simulink model "Udan_SOC"  (R2017b)
settings: Solver=FixedStepAuto  StartTime=0.0  StopTime=1000  FixedStep=0.1  RelTol=1e-3
values from neighbouring files (symbols this model uses):
  DenominatorOfIntegratorFactor = 100.0    [SOC_Stateflow.sldd]
  SOC_CalcSohLKT = 1.0    [SOC_Stateflow.sldd]
  SOC_CalcSOHTempLimit = 70.0    [SOC_Stateflow.sldd]
  SOC_CapPerCycle = 100.0    [SOC_Stateflow.sldd]
  SOC_CapTemp_HLimit = 200.0    [SOC_Stateflow.sldd]
  SOC_CapTemp_LLimit = 0.0    [SOC_Stateflow.sldd]
  Soc_ConfigInfo = 0    [SOC_Stateflow.sldd]
  SOC_DchgEndCalib = 0.0    [SOC_Stateflow.sldd]
  SOC_DiffVoltMin = 10.0    [SOC_Stateflow.sldd]
  SOC_DSOCJumpMax = 500.0    [SOC_Stateflow.sldd]
  SOC_EfficientHighLimit = 250.0    [SOC_Stateflow.sldd]
  SOC_EfficientLowLimit = 40.0    [SOC_Stateflow.sldd]
  SOC_EmptyAus = 0.0    [SOC_Stateflow.sldd]
  SOC_EnableOcv = 1.0    [SOC_Stateflow.sldd]
  SOC_END_CALIB_STATE : value not decoded    [SOC_Stateflow.sldd]
  SOC_HighRealSoc = 95.0    [SOC_Stateflow.sldd]
  SOC_LKTSohCycles = 0.0 1.0 10.0 20.0 30.0 40.0 50.0 60.0 70.0 80.0 90.0 100.0 110.0 120.0 130.0 140.0 150.0 160.0 170.0 180.0 190.0 200.0 210.0 220.0 230.0 240.0 250.0 260.0 270.0 280.0 290.0 300.0 310.0 320.0 330.0 340.0 350.0 360.0 370.0 380.0 390.0 400.0 410.0 420.0 430.0 440.0 450.0 460.0 470.0 480.0 490.0 500.0 510.0 520.0 530.0 540.0 550.0 560.0 570.0 580.0 590.0 600.0 610.0 620.0 630.0 640.0 650.0 660.0 670.0    [SOC_Stateflow.sldd]
  SOC_LKTSohTable = 1000.0 991.0 989.0 992.0 993.0 995.0 994.0 993.0 1000.0 997.0 1002.0 1000.0 992.0 1000.0 989.0 992.0 989.0 994.0 989.0 993.0 994.0 994.0 994.0 993.0 991.0 991.0 992.0 993.0 991.0 985.0 985.0 985.0 979.0 975.0 978.0 984.0 982.0 974.0 975.0 972.0 972.0 975.0 977.0 977.0 974.0 971.0 973.0 971.0 966.0 968.0 965.0 959.0 957.0 956.0 957.0 954.0 955.0 951.0 954.0 951.0 942.0 942.0 940.0 942.0 947.0 949.0    [SOC_Stateflow.sldd]
  SOC_LowRealSoc = 5.0    [SOC_Stateflow.sldd]
  SOC_NominalCap_AmS = 576000000.0    [SOC_Stateflow.sldd]
  SOC_NominalVol = 4000.0    [SOC_Stateflow.sldd]
  SOC_OCVTemp_HLimit = 106.0    [SOC_Stateflow.sldd]
  SOC_OCVTemp_LLimit = 29.0    [SOC_Stateflow.sldd]
  SOC_ShortCalibDSoc = 1.0    [SOC_Stateflow.sldd]
  SOC_SOCResolution = 10000.0    [SOC_Stateflow.sldd]
  SOC_SohCalcCapPercent = 8.0    [SOC_Stateflow.sldd]
  SOC_SohCalcHighLimit = 60.0    [SOC_Stateflow.sldd]
  SOC_SohCalcLowLimit = 10.0    [SOC_Stateflow.sldd]
  SOC_SohCalcMidLimit = 30.0    [SOC_Stateflow.sldd]
  SOC_SOHResolution = 1000.0    [SOC_Stateflow.sldd]
  SOC_State = <binary blob, 1163 chars, not shown>    [SOC_Stateflow.sldd]
  SOC_TempCap_CapBuffer : value not decoded    [SOC_Stateflow.sldd]
  SOC_TempCap_TempBuffer : value not decoded    [SOC_Stateflow.sldd]
  SocOcvCalib_ConfigInfo = 0.0    [SOC_Stateflow.sldd]
  SocOcvCalib_SocBuffer1 : value not decoded    [SOC_Stateflow.sldd]
  SocOcvCalib_TempBuffer : value not decoded    [SOC_Stateflow.sldd]
  SocOcvCalib_VoltageBuffer1 = 3300.0 3303.0 3305.0 3307.0 3310.0 3311.0 3313.0 3314.0 3316.0 3317.0 3319.0 3320.0 3322.0 3323.0 3325.0 3322.0 3323.0 3325.0 3310.0 3313.0 3315.0 3317.0 3320.0 3321.0 3323.0 3324.0 3326.0 3327.0 3329.0 3330.0 3332.0 3333.0 3335.0 3332.0 3333.0 3335.0 3320.0 3323.0 3325.0 3327.0 3330.0 3331.0 3333.0 3334.0 3336.0 3337.0 3339.0 3340.0 3342.0 3343.0 3345.0 3342.0 3343.0 3345.0 3330.0 3333.0 3335.0 3    [SOC_Stateflow.sldd]
  SOHCalibCycle = 10.0    [SOC_Stateflow.sldd]
undefined symbols (not defined in the file or in its folder): DatetimeM_GetReturnType, ParameterM_EeepParaIndexType, Soc_CumuLativeTypeType, SOC_EgthTempChgValue, Soc_EnergyBuffer, SOC_FithTempChgValue, SOC_FstSlowTempChgValue, SOC_FstTempChgValue, SOC_FthTempChgValue, SOC_MaxCap_AmS, SOC_SethTempChgValue, SOC_SixTempChgValue, SOC_SndSlowTempChgValue, SOC_SndTempChgValue, SOC_TrdSlowTempChgValue, SOC_TrdTempChgValue, SocDiagCalib_NoCalibReasonType
libraries: simulink x138, hdlsllib x24, dspindex x4
(part 6 of 10)

== system Udan_SOC/SOC_Calculate/UdanSOCCalcn/CalcnLeftChargeTime/CalcLeftTime1 ==
  DLeftCap : Inport
  LowTemp : Inport  Port=2
  PackCur : Inport  Port=3
  TotalCap : Inport  Port=4
  HighTemp : Inport  Port=5
  Enable : EnablePort
  Bus Selector : BusSelector  OutputSignals=FstDecreaseCur,SndDecreaseCur,TrdDecreaseCur,LstDecreaseCur
  Bus Selector1 : BusSelector  OutputSignals=FstDecreaseCur,SndDecreaseCur,TrdDecreaseCur,LstDecreaseCur
  CalcLeftTime : Stateflow chart  TreatAsAtomicUnit=on
  Constant : Constant  Value=9490  OutDataTypeStr=uint16
  Constant1 : Constant  Value=9000  OutDataTypeStr=uint16
  Constant10 : Constant  Value=SOC_SOCResolution  OutDataTypeStr=uint16
  Constant11 : Constant  Value=65535  OutDataTypeStr=uint32
  Constant2 : Constant  Value=9500  OutDataTypeStr=uint16
  Constant3 : Constant  Value=SOC_FstSlowTempChgValue  OutDataTypeStr=Bus: SOC_ChgCurrentType
  Constant4 : Constant  Value=SOC_FstSlowTempChgValue  OutDataTypeStr=Bus: SOC_ChgCurrentType
  Constant5 : Constant  Value=SOC_SndSlowTempChgValue  OutDataTypeStr=Bus: SOC_ChgCurrentType
  Constant6 : Constant  Value=SOC_TrdSlowTempChgValue  OutDataTypeStr=Bus: SOC_ChgCurrentType
  Constant7 : Constant  Value=SOC_SndSlowTempChgValue  OutDataTypeStr=Bus: SOC_ChgCurrentType
  Constant8 : Constant  Value=SOC_TrdSlowTempChgValue  OutDataTypeStr=Bus: SOC_ChgCurrentType
  Constant9 : Constant  Value=65535  OutDataTypeStr=uint32
  Divide : Product  Inputs=*/*  OutDataTypeStr=uint32
  Divide1 : Product  Inputs=*/*  OutDataTypeStr=uint32
  Divide2 : Product  Inputs=*/*  OutDataTypeStr=uint32
  MinMax{,1..3} (4 alike) : MinMax  Inputs=2
  SelectChgCurrent : Stateflow chart  TreatAsAtomicUnit=on
  SelectChgCurrent1 : Stateflow chart  TreatAsAtomicUnit=on
  Terminator : Terminator
  Terminator1 : Terminator
  LeftChargeTime : Outport
  PackCurOk : Outport  Port=2
  wires:
  Constant/1 -> Divide/3
  Constant1/1 -> Divide1/3
  Constant10/1 -> Divide2/2, Divide1/2, Divide/2
  Constant2/1 -> Divide2/3
  LowTemp/1 -> SelectChgCurrent/1(BatTemp)
  Constant4/1 -> SelectChgCurrent/2(FstChgCur)
  Constant5/1 -> SelectChgCurrent/3(SndChgCur)
  Constant6/1 -> SelectChgCurrent/4(TrdChgCur)
  SelectChgCurrent/1(ChgCurOut) -> Bus Selector/1
  DLeftCap/1 -> CalcLeftTime/1(DleftCap)
  TotalCap/1 -> CalcLeftTime/3(NominalCap), Divide2/1, Divide1/1, Divide/1
  Divide/1 -> CalcLeftTime/4(FstDecPnt)
  Constant9/1 -> CalcLeftTime/5(SndDecPnt)
  Constant11/1 -> CalcLeftTime/6(TrdDecPnt)
  MinMax/1 -> CalcLeftTime/7(Cur1)
  MinMax1/1 -> CalcLeftTime/8(Cur2)
  MinMax2/1 -> CalcLeftTime/9(Cur3)
  MinMax3/1 -> CalcLeftTime/10(Cur4)
  CalcLeftTime/1(TimeOut) -> LeftChargeTime/1
  PackCur/1 -> CalcLeftTime/2(PackCur)
  CalcLeftTime/2(result) -> PackCurOk/1
  Constant8/1 -> SelectChgCurrent1/4(TrdChgCur)
  Constant3/1 -> SelectChgCurrent1/2(FstChgCur)
  Constant7/1 -> SelectChgCurrent1/3(SndChgCur)
  HighTemp/1 -> SelectChgCurrent1/1(BatTemp)
  SelectChgCurrent1/1(ChgCurOut) -> Bus Selector1/1
  Bus Selector1/1 -> [HighTemp_FstDecCur]  "<FstDecreaseCur>"
  Bus Selector1/2 -> [HighTemp_SndDecCur]  "<SndDecreaseCur>"
  Bus Selector1/3 -> [HighTemp_TrdDecCur]  "<TrdDecreaseCur>"
  Bus Selector1/4 -> [LstTemp_LastDecCur]  "<LstDecreaseCur>"
  Bus Selector/1 -> MinMax/1  "<FstDecreaseCur>"
  [HighTemp_FstDecCur] -> MinMax/2
  Bus Selector/2 -> MinMax1/1  "<SndDecreaseCur>"
  [HighTemp_SndDecCur] -> MinMax1/2
  Bus Selector/3 -> MinMax2/1  "<TrdDecreaseCur>"
  [HighTemp_TrdDecCur] -> MinMax2/2
  [LstTemp_LastDecCur] -> MinMax3/2
  Bus Selector/4 -> MinMax3/1  "<LstDecreaseCur>"
  Divide2/1 -> Terminator1/1
  Divide1/1 -> Terminator/1

== system Udan_SOC/SOC_Calculate/UdanSOCCalcn/CalcnLeftChargeTime/DiagDrop1 ==
  LeftChargeTimeOut : Inport
  NowTime : Inport  Port=2
  LastChargeTime : Inport  Port=3
  Enable : EnablePort
  Constant : Constant  Value=6  OutDataTypeStr=uint8
  Constant1 : Constant  Value=100  OutDataTypeStr=uint8
  Constant2 : Constant  Value=0  OutDataTypeStr=boolean
  Delay : Delay  DelayLength=1  InitialCondition=1
  DiagDropCore : Stateflow chart  TreatAsAtomicUnit=on
  Switch : Switch  Criteria=u2 > Threshold  OutDataTypeStr=uint32
  Unit Delay1 : UnitDelay  SampleTime=-1
  Unit Delay2 : UnitDelay  SampleTime=-1
  LeftCahrgeTime : Outport
  wires:
  LastChargeTime/1 -> DiagDropCore/6(LastCurrentSend)
  DiagDropCore/1(CurrentSend) -> Switch/3  "CurrentSend"
  [CurrentOut] -> Switch/1
  Constant2/1 -> Delay/1
  Delay/1 -> Switch/2
  Constant1/1 -> DiagDropCore/5(OutUpdateTick)
  Constant/1 -> DiagDropCore/4(increaseStep), DiagDropCore/3(decreaseStep)
  LeftChargeTimeOut/1 -> DiagDropCore/1(CurrentOut), [CurrentOut]
  NowTime/1 -> DiagDropCore/2(NowTime)
  DiagDropCore/2(CurState) -> Unit Delay2/1  "CurState"
  DiagDropCore/3(CurTime) -> Unit Delay1/1
  Unit Delay1/1 -> DiagDropCore/8(LastTime)
  Unit Delay2/1 -> DiagDropCore/7(LastState)
  Switch/1 -> LeftCahrgeTime/1

== system Udan_SOC/SOC_Calculate/UdanSOCCalcn/CalcnLeftChargeTime/Triggered Subsystem ==
  In1 : Inport
  Trigger : TriggerPort  VariantControl=Variant
  Out1 : Outport
  wires:
  In1/1 -> Out1/1

== system Udan_SOC/SOC_Calculate/UdanSOCCalcn/CalcnLeftChargeTime/Triggered Subsystem1 ==
  In1 : Inport
  Trigger : TriggerPort  VariantControl=Variant
  Out1 : Outport
  wires:
  In1/1 -> Out1/1

== system Udan_SOC/SOC_Calculate/UdanSOCCalcn/CalcnLeftChargeTime/Triggered Subsystem4 ==
  Trigger : TriggerPort  VariantControl=Variant
  Constant : Constant  OutDataTypeStr=boolean
  Data Store Write : DataStoreWrite  DataStoreName=SmoothEnable
  wires:
  Constant/1 -> Data Store Write/1

== system Udan_SOC/SOC_Calculate/UdanSOCCalcn/CalibEmptySOC/ConvertSOC2AH ==
  BatTemp : Inport
  SOC : Inport  Port=2
  SOH : Inport  Port=3
  Add3 : Sum  Inputs=+-
  Add5 : Sum  AccumDataTypeStr=int32  OutDataTypeStr=int32
  Constant : Constant  Value=0  OutDataTypeStr=uint8
  Constant1 : Constant  Value=SOC_NominalCap_AmS
  Constant22 : Constant  Value=SOC_SOCResolution  OutDataTypeStr=uint16
  Constant24 : Constant  Value=SOC_SOHResolution  OutDataTypeStr=uint16
  Constant25 : Constant  Value=SOC_NominalCap_AmS
  Constant26 : Constant  Value=SOC_SOHResolution  OutDataTypeStr=uint16
  Constant31 : Constant  Value=SOC_NominalCap_AmS
  Constant42 : Constant  Value=SOC_SOHResolution  OutDataTypeStr=uint16
  Constant43 : Constant  Value=SOC_TempCap_CapBuffer
  Divide16 : Product  Inputs=*/*  OutDataTypeStr=uint32
  Divide3 : Product  Inputs=*/*  OutDataTypeStr=uint32
  Divide4 : Product  Inputs=**  OutDataTypeStr=int32
  Divide5 : Product  Inputs=**  OutDataTypeStr=uint32
  Divide6 : Product  Inputs=*/  OutDataTypeStr=int32
  Divide8 : Product  Inputs=*/  OutDataTypeStr=uint32
  MinMax : MinMax  Function=max
  MinMax1 : MinMax  Function=max  Inputs=2
  Saturation Dynamic : simulink/Discontinuities/Saturation Dynamic  OutMin=[]  OutMax=[]  OutDataTypeStr=Inherit: Same as second input  OutDataType=fixdt(1, 16)  OutScaling=2^-10  DoSatur=off
  TempCapTable1 : Lookup_n-D  NumberOfTableDimensions=1  BreakpointsForDimension1=SOC_TempCap_TempBuffer  Table=SOC_TempCap_CapBuffer  ExtrapMethod=Clip  InternalRulePriority=Speed  OutDataTypeStr=uint16  RndMeth=Simplest  InputSameDT=on
  AHOut : Outport
  wires:
  Add5/1 -> Divide3/1
  Divide4/1 -> Add5/2
  SOH/1 -> Divide3/3
  BatTemp/1 -> TempCapTable1/1
  SOC/1 -> Divide4/2
  Divide3/1 -> AHOut/1
  Divide6/1 -> Divide4/1
  Saturation Dynamic/1 -> Divide6/1, Add3/2
  Constant26/1 -> Divide3/2
  Constant24/1 -> Divide8/2
  Constant22/1 -> Divide6/2
  Constant1/1 -> Divide8/1
  MinMax1/1 -> Add3/1, Saturation Dynamic/1
  Add3/1 -> Add5/1
  TempCapTable1/1 -> Divide5/1
  Divide8/1 -> Divide5/2
  Divide5/1 -> Saturation Dynamic/2
  Constant/1 -> Saturation Dynamic/3
  Constant42/1 -> Divide16/2
  Constant43/1 -> MinMax/1
  MinMax/1 -> Divide16/3
  Divide16/1 -> MinMax1/1
  Constant25/1 -> MinMax1/2
  Constant31/1 -> Divide16/1

== system Udan_SOC/SOC_Calculate/UdanSOCCalcn/CalibFullSOC/Subsystem ==
  data : Inport
  HighIndex : Inport  Port=2
  LowIndex : Inport  Port=3
  Bit Rotate : hdlsllib/Logic and Bit Operations/Bit Rotate  mode=Rotate Right  N=16
      settings: SourceProductName=HDL Coder  SourceProductBaseCode=HD
  Data Type Conversion : DataTypeConversion  OutDataTypeStr=uint16
  Data Type Conversion1 : DataTypeConversion  OutDataTypeStr=uint16
  S-Function : S-Function  FunctionName=sfn_NVMWrite  SFunctionDeploymentMode=off  EnableBusSupport=off
  S-Function1 : S-Function  FunctionName=sfn_NVMWrite  SFunctionDeploymentMode=off  EnableBusSupport=off
  Terminator : Terminator
  Terminator1 : Terminator
  wires:
  data/1 -> Data Type Conversion1/1, Bit Rotate/1
  Data Type Conversion/1 -> S-Function/2
  S-Function1/1 -> Terminator1/1
  Bit Rotate/1 -> Data Type Conversion/1
  Data Type Conversion1/1 -> S-Function1/2
  S-Function/1 -> Terminator/1
  HighIndex/1 -> S-Function/1
  LowIndex/1 -> S-Function1/1

== system Udan_SOC/SOC_Calculate/UdanSOCCalcn/CapAdder1/ConvertSOC2AH ==
  BatTemp : Inport
  SOC : Inport  Port=2
  SOH : Inport  Port=3
  Add3 : Sum  Inputs=+-
  Add5 : Sum  AccumDataTypeStr=int32  OutDataTypeStr=int32
  Constant : Constant  Value=0  OutDataTypeStr=uint8
  Constant1 : Constant  Value=SOC_NominalCap_AmS
  Constant22 : Constant  Value=SOC_SOCResolution  OutDataTypeStr=uint16
  Constant24 : Constant  Value=SOC_SOHResolution  OutDataTypeStr=uint16
  Constant25 : Constant  Value=SOC_NominalCap_AmS
  Constant26 : Constant  Value=SOC_SOHResolution  OutDataTypeStr=uint16
  Constant31 : Constant  Value=SOC_NominalCap_AmS
  Constant42 : Constant  Value=SOC_SOHResolution  OutDataTypeStr=uint16
  Constant43 : Constant  Value=SOC_TempCap_CapBuffer
  Divide16 : Product  Inputs=*/*  OutDataTypeStr=uint32
  Divide3 : Product  Inputs=*/*  OutDataTypeStr=uint32
  Divide4 : Product  Inputs=**  OutDataTypeStr=int32
  Divide5 : Product  Inputs=**  OutDataTypeStr=uint32
  Divide6 : Product  Inputs=*/  OutDataTypeStr=int32
  Divide8 : Product  Inputs=*/  OutDataTypeStr=uint32
  MinMax : MinMax  Function=max
  MinMax1 : MinMax  Function=max  Inputs=2
  Saturation Dynamic : simulink/Discontinuities/Saturation Dynamic  OutMin=[]  OutMax=[]  OutDataTypeStr=Inherit: Same as second input  OutDataType=fixdt(1, 16)  OutScaling=2^-10  DoSatur=off
  TempCapTable1 : Lookup_n-D  NumberOfTableDimensions=1  BreakpointsForDimension1=SOC_TempCap_TempBuffer  Table=SOC_TempCap_CapBuffer  ExtrapMethod=Clip  InternalRulePriority=Speed  OutDataTypeStr=uint16  RndMeth=Simplest  InputSameDT=on
  AHOut : Outport
  NoUsedCap : Outport  Port=2
  Tcap : Outport  Port=3
  wires:
  Add5/1 -> Divide3/1
  Divide4/1 -> Add5/2
  SOH/1 -> Divide3/3
  BatTemp/1 -> TempCapTable1/1
  SOC/1 -> Divide4/2
  Divide3/1 -> AHOut/1
  Divide6/1 -> Divide4/1
  Saturation Dynamic/1 -> Tcap/1, Divide6/1, Add3/2
  Constant26/1 -> Divide3/2
  Constant24/1 -> Divide8/2
  Constant22/1 -> Divide6/2
  Constant1/1 -> Divide8/1
  MinMax1/1 -> Saturation Dynamic/1, Add3/1
  Add3/1 -> NoUsedCap/1, Add5/1
  TempCapTable1/1 -> Divide5/1
  Divide8/1 -> Divide5/2
  Divide5/1 -> Saturation Dynamic/2
  Constant/1 -> Saturation Dynamic/3
  Constant42/1 -> Divide16/2
  Constant25/1 -> MinMax1/2
  Divide16/1 -> MinMax1/1
  MinMax/1 -> Divide16/3
  Constant43/1 -> MinMax/1
  Constant31/1 -> Divide16/1

== system Udan_SOC/SOC_Calculate/UdanSOCCalcn/CapAdder1/ConvertSOC2AH1 ==
  BatTemp : Inport
  SOC : Inport  Port=2
  SOH : Inport  Port=3
  Add3 : Sum  Inputs=+-
  Add5 : Sum  AccumDataTypeStr=int32  OutDataTypeStr=int32
  Constant : Constant  Value=0  OutDataTypeStr=uint8
  Constant1 : Constant  Value=SOC_NominalCap_AmS
  Constant22 : Constant  Value=SOC_SOCResolution  OutDataTypeStr=uint16
  Constant24 : Constant  Value=SOC_SOHResolution  OutDataTypeStr=uint16
  Constant25 : Constant  Value=SOC_NominalCap_AmS
  Constant26 : Constant  Value=SOC_SOHResolution  OutDataTypeStr=uint16
  Constant31 : Constant  Value=SOC_NominalCap_AmS
  Constant42 : Constant  Value=SOC_SOHResolution  OutDataTypeStr=uint16
  Constant43 : Constant  Value=SOC_TempCap_CapBuffer
  Divide16 : Product  Inputs=*/*  OutDataTypeStr=uint32
  Divide3 : Product  Inputs=*/*  OutDataTypeStr=uint32
  Divide4 : Product  Inputs=**  OutDataTypeStr=int32
  Divide5 : Product  Inputs=**  OutDataTypeStr=uint32
  Divide6 : Product  Inputs=*/  OutDataTypeStr=int32
  Divide8 : Product  Inputs=*/  OutDataTypeStr=uint32
  MinMax : MinMax  Function=max
  MinMax1 : MinMax  Function=max  Inputs=2
  Saturation Dynamic : simulink/Discontinuities/Saturation Dynamic  OutMin=[]  OutMax=[]  OutDataTypeStr=Inherit: Same as second input  OutDataType=fixdt(1, 16)  OutScaling=2^-10  DoSatur=off
  TempCapTable1 : Lookup_n-D  NumberOfTableDimensions=1  BreakpointsForDimension1=SOC_TempCap_TempBuffer  Table=SOC_TempCap_CapBuffer  ExtrapMethod=Clip  InternalRulePriority=Speed  OutDataTypeStr=uint16  RndMeth=Simplest  InputSameDT=on
  AHOut : Outport
  wires:
  Add5/1 -> Divide3/1
  Divide4/1 -> Add5/2
  SOH/1 -> Divide3/3
  BatTemp/1 -> TempCapTable1/1
  SOC/1 -> Divide4/2
  Divide3/1 -> AHOut/1
  Divide6/1 -> Divide4/1
  Saturation Dynamic/1 -> Divide6/1, Add3/2
  Constant26/1 -> Divide3/2
  Constant24/1 -> Divide8/2
  Constant22/1 -> Divide6/2
  Constant1/1 -> Divide8/1
  MinMax1/1 -> Add3/1, Saturation Dynamic/1
  Add3/1 -> Add5/1
  TempCapTable1/1 -> Divide5/1
  Divide8/1 -> Divide5/2
  Divide5/1 -> Saturation Dynamic/2
  Constant/1 -> Saturation Dynamic/3
  Constant31/1 -> Divide16/1
  MinMax/1 -> Divide16/3
  Divide16/1 -> MinMax1/1
  Constant25/1 -> MinMax1/2
  Constant42/1 -> Divide16/2
  Constant43/1 -> MinMax/1

== system Udan_SOC/SOC_Calculate/UdanSOCCalcn/CapAdder1/ConvertSOC2AH2 ==
  BatTemp : Inport
  SOC : Inport  Port=2
  SOH : Inport  Port=3
  Add3 : Sum  Inputs=+-
  Add5 : Sum  AccumDataTypeStr=int32  OutDataTypeStr=int32
  Constant : Constant  Value=0  OutDataTypeStr=uint8
  Constant1 : Constant  Value=SOC_NominalCap_AmS
  Constant22 : Constant  Value=SOC_SOCResolution  OutDataTypeStr=uint16
  Constant24 : Constant  Value=SOC_SOHResolution  OutDataTypeStr=uint16
  Constant25 : Constant  Value=SOC_NominalCap_AmS
  Constant26 : Constant  Value=SOC_SOHResolution  OutDataTypeStr=uint16
  Constant31 : Constant  Value=SOC_NominalCap_AmS
  Constant42 : Constant  Value=SOC_SOHResolution  OutDataTypeStr=uint16
  Constant43 : Constant  Value=SOC_TempCap_CapBuffer
  Divide16 : Product  Inputs=*/*  OutDataTypeStr=uint32
  Divide3 : Product  Inputs=*/*  OutDataTypeStr=uint32
  Divide4 : Product  Inputs=**  OutDataTypeStr=int32
  Divide5 : Product  Inputs=**  OutDataTypeStr=uint32
  Divide6 : Product  Inputs=*/  OutDataTypeStr=int32
  Divide8 : Product  Inputs=*/  OutDataTypeStr=uint32
  MinMax : MinMax  Function=max
  MinMax1 : MinMax  Function=max  Inputs=2
  Saturation Dynamic : simulink/Discontinuities/Saturation Dynamic  OutMin=[]  OutMax=[]  OutDataTypeStr=Inherit: Same as second input  OutDataType=fixdt(1, 16)  OutScaling=2^-10  DoSatur=off
  TempCapTable1 : Lookup_n-D  NumberOfTableDimensions=1  BreakpointsForDimension1=SOC_TempCap_TempBuffer  Table=SOC_TempCap_CapBuffer  ExtrapMethod=Clip  InternalRulePriority=Speed  OutDataTypeStr=uint16  RndMeth=Simplest  InputSameDT=on
  AHOut : Outport
  wires:
  Add5/1 -> Divide3/1
  Divide4/1 -> Add5/2
  SOH/1 -> Divide3/3
  BatTemp/1 -> TempCapTable1/1
  SOC/1 -> Divide4/2
  Divide3/1 -> AHOut/1
  Divide6/1 -> Divide4/1
  Saturation Dynamic/1 -> Divide6/1, Add3/2
  Constant26/1 -> Divide3/2
  Constant24/1 -> Divide8/2
  Constant22/1 -> Divide6/2
  Constant1/1 -> Divide8/1
  MinMax1/1 -> Add3/1, Saturation Dynamic/1
  Add3/1 -> Add5/1
  TempCapTable1/1 -> Divide5/1
  Divide8/1 -> Divide5/2
  Divide5/1 -> Saturation Dynamic/2
  Constant/1 -> Saturation Dynamic/3
  Constant31/1 -> Divide16/1
  MinMax/1 -> Divide16/3
  Divide16/1 -> MinMax1/1
  Constant25/1 -> MinMax1/2
  Constant42/1 -> Divide16/2
  Constant43/1 -> MinMax/1

== system Udan_SOC/SOC_Calculate/UdanSOCCalcn/CapAdder1/ConvertSOC2AH3 ==
  BatTemp : Inport
  SOC : Inport  Port=2
  SOH : Inport  Port=3
  Add3 : Sum  Inputs=+-
  Add5 : Sum  AccumDataTypeStr=int32  OutDataTypeStr=int32
  Constant : Constant  Value=0  OutDataTypeStr=uint8
  Constant1 : Constant  Value=SOC_NominalCap_AmS
  Constant22 : Constant  Value=SOC_SOCResolution  OutDataTypeStr=uint16
  Constant24 : Constant  Value=SOC_SOHResolution  OutDataTypeStr=uint16
  Constant25 : Constant  Value=SOC_NominalCap_AmS
  Constant26 : Constant  Value=SOC_SOHResolution  OutDataTypeStr=uint16
  Constant31 : Constant  Value=SOC_NominalCap_AmS
  Constant42 : Constant  Value=SOC_SOHResolution  OutDataTypeStr=uint16
  Constant43 : Constant  Value=SOC_TempCap_CapBuffer
  Divide16 : Product  Inputs=*/*  OutDataTypeStr=uint32
  Divide3 : Product  Inputs=*/*  OutDataTypeStr=uint32
  Divide4 : Product  Inputs=**  OutDataTypeStr=int32
  Divide5 : Product  Inputs=**  OutDataTypeStr=uint32
  Divide6 : Product  Inputs=*/  OutDataTypeStr=int32
  Divide8 : Product  Inputs=*/  OutDataTypeStr=uint32
  MinMax : MinMax  Function=max
  MinMax1 : MinMax  Function=max  Inputs=2
  Saturation Dynamic : simulink/Discontinuities/Saturation Dynamic  OutMin=[]  OutMax=[]  OutDataTypeStr=Inherit: Same as second input  OutDataType=fixdt(1, 16)  OutScaling=2^-10  DoSatur=off
  TempCapTable1 : Lookup_n-D  NumberOfTableDimensions=1  BreakpointsForDimension1=SOC_TempCap_TempBuffer  Table=SOC_TempCap_CapBuffer  ExtrapMethod=Clip  InternalRulePriority=Speed  OutDataTypeStr=uint16  RndMeth=Simplest  InputSameDT=on
  AHOut : Outport
  wires:
  Add5/1 -> Divide3/1
  Divide4/1 -> Add5/2
  SOH/1 -> Divide3/3
  BatTemp/1 -> TempCapTable1/1
  SOC/1 -> Divide4/2
  Divide3/1 -> AHOut/1
  Divide6/1 -> Divide4/1
  Saturation Dynamic/1 -> Divide6/1, Add3/2
  Constant26/1 -> Divide3/2
  Constant24/1 -> Divide8/2
  Constant22/1 -> Divide6/2
  Constant1/1 -> Divide8/1
  MinMax1/1 -> Add3/1, Saturation Dynamic/1
  Add3/1 -> Add5/1
  TempCapTable1/1 -> Divide5/1
  Divide8/1 -> Divide5/2
  Divide5/1 -> Saturation Dynamic/2
  Constant/1 -> Saturation Dynamic/3
  Constant31/1 -> Divide16/1
  MinMax/1 -> Divide16/3
  Divide16/1 -> MinMax1/1
  Constant25/1 -> MinMax1/2
  Constant42/1 -> Divide16/2
  Constant43/1 -> MinMax/1

== system Udan_SOC/SOC_Calculate/UdanSOCCalcn/CapAdder1/ConvertSOC2AH4 ==
  BatTemp : Inport
  SOC : Inport  Port=2
  SOH : Inport  Port=3
  Add3 : Sum  Inputs=+-
  Add5 : Sum  AccumDataTypeStr=int32  OutDataTypeStr=int32
  Constant : Constant  Value=0  OutDataTypeStr=uint8
  Constant1 : Constant  Value=SOC_NominalCap_AmS
  Constant22 : Constant  Value=SOC_SOCResolution  OutDataTypeStr=uint16
  Constant24 : Constant  Value=SOC_SOHResolution  OutDataTypeStr=uint16
  Constant25 : Constant  Value=SOC_NominalCap_AmS
  Constant26 : Constant  Value=SOC_SOHResolution  OutDataTypeStr=uint16
  Constant31 : Constant  Value=SOC_NominalCap_AmS
  Constant42 : Constant  Value=SOC_SOHResolution  OutDataTypeStr=uint16
  Constant43 : Constant  Value=SOC_TempCap_CapBuffer
  Divide16 : Product  Inputs=*/*  OutDataTypeStr=uint32
  Divide3 : Product  Inputs=*/*  OutDataTypeStr=uint32
  Divide4 : Product  Inputs=**  OutDataTypeStr=int32
  Divide5 : Product  Inputs=**  OutDataTypeStr=uint32
  Divide6 : Product  Inputs=*/  OutDataTypeStr=int32
  Divide8 : Product  Inputs=*/  OutDataTypeStr=uint32
  MinMax : MinMax  Function=max
  MinMax1 : MinMax  Function=max  Inputs=2
  Saturation Dynamic : simulink/Discontinuities/Saturation Dynamic  OutMin=[]  OutMax=[]  OutDataTypeStr=Inherit: Same as second input  OutDataType=fixdt(1, 16)  OutScaling=2^-10  DoSatur=off
  TempCapTable1 : Lookup_n-D  NumberOfTableDimensions=1  BreakpointsForDimension1=SOC_TempCap_TempBuffer  Table=SOC_TempCap_CapBuffer  ExtrapMethod=Clip  InternalRulePriority=Speed  OutDataTypeStr=uint16  RndMeth=Simplest  InputSameDT=on
  AHOut : Outport
  wires:
  Add5/1 -> Divide3/1
  Divide4/1 -> Add5/2
  SOH/1 -> Divide3/3
  BatTemp/1 -> TempCapTable1/1
  SOC/1 -> Divide4/2
  Divide3/1 -> AHOut/1
  Divide6/1 -> Divide4/1
  Saturation Dynamic/1 -> Divide6/1, Add3/2
  Constant26/1 -> Divide3/2
  Constant24/1 -> Divide8/2
  Constant22/1 -> Divide6/2
  Constant1/1 -> Divide8/1
  MinMax1/1 -> Add3/1, Saturation Dynamic/1
  Add3/1 -> Add5/1
  TempCapTable1/1 -> Divide5/1
  Divide8/1 -> Divide5/2
  Divide5/1 -> Saturation Dynamic/2
  Constant/1 -> Saturation Dynamic/3
  Constant31/1 -> Divide16/1
  MinMax/1 -> Divide16/3
  Divide16/1 -> MinMax1/1
  Constant25/1 -> MinMax1/2
  Constant42/1 -> Divide16/2
  Constant43/1 -> MinMax/1

== system Udan_SOC/SOC_Calculate/UdanSOCCalcn/CapAdder1/ConvertSOC2AH5 ==
  BatTemp : Inport
  SOC : Inport  Port=2
  SOH : Inport  Port=3
  Add3 : Sum  Inputs=+-
  Add5 : Sum  AccumDataTypeStr=int32  OutDataTypeStr=int32
  Constant : Constant  Value=0  OutDataTypeStr=uint8
  Constant1 : Constant  Value=SOC_NominalCap_AmS
  Constant22 : Constant  Value=SOC_SOCResolution  OutDataTypeStr=uint16
  Constant24 : Constant  Value=SOC_SOHResolution  OutDataTypeStr=uint16
  Constant25 : Constant  Value=SOC_NominalCap_AmS
  Constant26 : Constant  Value=SOC_SOHResolution  OutDataTypeStr=uint16
  Constant31 : Constant  Value=SOC_NominalCap_AmS
  Constant42 : Constant  Value=SOC_SOHResolution  OutDataTypeStr=uint16
  Constant43 : Constant  Value=SOC_TempCap_CapBuffer
  Divide16 : Product  Inputs=*/*  OutDataTypeStr=uint32
  Divide3 : Product  Inputs=*/*  OutDataTypeStr=uint32
  Divide4 : Product  Inputs=**  OutDataTypeStr=int32
  Divide5 : Product  Inputs=**  OutDataTypeStr=uint32
  Divide6 : Product  Inputs=*/  OutDataTypeStr=int32
  Divide8 : Product  Inputs=*/  OutDataTypeStr=uint32
  MinMax : MinMax  Function=max
  MinMax1 : MinMax  Function=max  Inputs=2
  Saturation Dynamic : simulink/Discontinuities/Saturation Dynamic  OutMin=[]  OutMax=[]  OutDataTypeStr=Inherit: Same as second input  OutDataType=fixdt(1, 16)  OutScaling=2^-10  DoSatur=off
  TempCapTable1 : Lookup_n-D  NumberOfTableDimensions=1  BreakpointsForDimension1=SOC_TempCap_TempBuffer  Table=SOC_TempCap_CapBuffer  ExtrapMethod=Clip  InternalRulePriority=Speed  OutDataTypeStr=uint16  RndMeth=Simplest  InputSameDT=on
  AHOut : Outport
  wires:
  Add5/1 -> Divide3/1
  Divide4/1 -> Add5/2
  SOH/1 -> Divide3/3
  BatTemp/1 -> TempCapTable1/1
  SOC/1 -> Divide4/2
  Divide3/1 -> AHOut/1
  Divide6/1 -> Divide4/1
  Saturation Dynamic/1 -> Divide6/1, Add3/2
  Constant26/1 -> Divide3/2
  Constant24/1 -> Divide8/2
  Constant22/1 -> Divide6/2
  Constant1/1 -> Divide8/1
  MinMax1/1 -> Add3/1, Saturation Dynamic/1
  Add3/1 -> Add5/1
  TempCapTable1/1 -> Divide5/1
  Divide8/1 -> Divide5/2
  Divide5/1 -> Saturation Dynamic/2
  Constant/1 -> Saturation Dynamic/3
  Constant31/1 -> Divide16/1
  MinMax/1 -> Divide16/3
  Divide16/1 -> MinMax1/1
  Constant25/1 -> MinMax1/2
  Constant42/1 -> Divide16/2
  Constant43/1 -> MinMax/1

== system Udan_SOC/SOC_Calculate/UdanSOCCalcn/CapAdder1/ConvertSOC2AH6 ==
  BatTemp : Inport
  SOC : Inport  Port=2
  SOH : Inport  Port=3
  Add3 : Sum  Inputs=+-
  Add5 : Sum  AccumDataTypeStr=int32  OutDataTypeStr=int32
  Constant : Constant  Value=0  OutDataTypeStr=uint8
  Constant1 : Constant  Value=SOC_NominalCap_AmS
  Constant22 : Constant  Value=SOC_SOCResolution  OutDataTypeStr=uint16
  Constant24 : Constant  Value=SOC_SOHResolution  OutDataTypeStr=uint16
  Constant25 : Constant  Value=SOC_NominalCap_AmS
  Constant26 : Constant  Value=SOC_SOHResolution  OutDataTypeStr=uint16
  Constant31 : Constant  Value=SOC_NominalCap_AmS
  Constant42 : Constant  Value=SOC_SOHResolution  OutDataTypeStr=uint16
  Constant43 : Constant  Value=SOC_TempCap_CapBuffer
  Divide16 : Product  Inputs=*/*  OutDataTypeStr=uint32
  Divide3 : Product  Inputs=*/*  OutDataTypeStr=uint32
  Divide4 : Product  Inputs=**  OutDataTypeStr=int32
  Divide5 : Product  Inputs=**  OutDataTypeStr=uint32
  Divide6 : Product  Inputs=*/  OutDataTypeStr=int32
  Divide8 : Product  Inputs=*/  OutDataTypeStr=uint32
  MinMax : MinMax  Function=max
  MinMax1 : MinMax  Function=max  Inputs=2
  Saturation Dynamic : simulink/Discontinuities/Saturation Dynamic  OutMin=[]  OutMax=[]  OutDataTypeStr=Inherit: Same as second input  OutDataType=fixdt(1, 16)  OutScaling=2^-10  DoSatur=off
  TempCapTable1 : Lookup_n-D  NumberOfTableDimensions=1  BreakpointsForDimension1=SOC_TempCap_TempBuffer  Table=SOC_TempCap_CapBuffer  ExtrapMethod=Clip  InternalRulePriority=Speed  OutDataTypeStr=uint16  RndMeth=Simplest  InputSameDT=on
  AHOut : Outport
  wires:
  Add5/1 -> Divide3/1
  Divide4/1 -> Add5/2
  SOH/1 -> Divide3/3
  BatTemp/1 -> TempCapTable1/1
  SOC/1 -> Divide4/2
  Divide3/1 -> AHOut/1
  Divide6/1 -> Divide4/1
  Saturation Dynamic/1 -> Divide6/1, Add3/2
  Constant26/1 -> Divide3/2
  Constant24/1 -> Divide8/2
  Constant22/1 -> Divide6/2
  Constant1/1 -> Divide8/1
  MinMax1/1 -> Add3/1, Saturation Dynamic/1
  Add3/1 -> Add5/1
  TempCapTable1/1 -> Divide5/1
  Divide8/1 -> Divide5/2
  Divide5/1 -> Saturation Dynamic/2
  Constant/1 -> Saturation Dynamic/3
  Constant31/1 -> Divide16/1
  MinMax/1 -> Divide16/3
  Divide16/1 -> MinMax1/1
  Constant25/1 -> MinMax1/2
  Constant42/1 -> Divide16/2
  Constant43/1 -> MinMax/1

== system Udan_SOC/SOC_Calculate/UdanSOCCalcn/CapAdder1/Enabled Subsystem1 ==
  CalculatedSOC : Inport
  Current : Inport  Port=2
  CellLowTemp : Inport  Port=3
  UCell : Inport  Port=4
  soh : Inport  Port=5
  Enable : EnablePort
  Chart : Stateflow chart  TreatAsAtomicUnit=on
  Constant : Constant  Value=4  OutDataTypeStr=uint8
  Enabled Subsystem1 : Subsystem  TreatAsAtomicUnit=on
  Enumerated Constant : simulink/Sources/Enumerated Constant  OutDataTypeStr=Enum: SOC_END_CALIB_STATE  Value=SOC_END_CALIB_STATE.SOC_STATE_CALCNSOC  SampleTime=inf
      settings: SourceProductName=Simulink
  Function-Call Subsystem : Subsystem  Commented=on  TreatAsAtomicUnit=on
  Logical Operator : Logic  Operator=NOT  AllPortsSameDT=off  OutDataTypeStr=boolean
  Relational Operator : RelationalOperator  Operator===  OutDataTypeStr=boolean  RndMeth=Simplest
  Relational Operator1 : RelationalOperator  Operator=<=  OutDataTypeStr=boolean  RndMeth=Simplest
  Switch : Switch  Criteria=u2 > Threshold
  Switch1 : Switch  Criteria=u2 > Threshold
  SOCOut : Outport
  wires:
  Chart/1(Start_SOC) -> Relational Operator/1
  Relational Operator/1 -> Switch/2, Logical Operator/1
  Enumerated Constant/1 -> Relational Operator/2
  CalculatedSOC/1 -> [CalculatedSOC], Switch/1
  Switch/1 -> SOCOut/1
  Logical Operator/1 -> Enabled Subsystem1/Enable
  Enabled Subsystem1/2(LeftCap2) -> Switch1/3
  Current/1 -> Chart/1(Current)
  CellLowTemp/1 -> Enabled Subsystem1/1(CellLowTemp)
  UCell/1 -> Enabled Subsystem1/2(UCell)
  Enabled Subsystem1/1(LKTSOC) -> Relational Operator1/1
  Constant/1 -> Relational Operator1/2
  Relational Operator1/1 -> Switch1/2
  [CalculatedSOC] -> Switch1/1
  Switch1/1 -> Switch/3
  Chart/2(SetLowPower()) -> Function-Call Subsystem/Trigger
  [CalculatedSOC] -> Enabled Subsystem1/3(CalcSoc)
  soh/1 -> Enabled Subsystem1/4(soh)

== system Udan_SOC/SOC_Calculate/UdanSOCCalcn/CapAdder1/Function-Call Subsystem ==
  LeftCapIn : Inport
  function : TriggerPort  VariantControl=Variant
  LeftCapOut : Outport
  wires:
  LeftCapIn/1 -> LeftCapOut/1

== system Udan_SOC/SOC_Calculate/UdanSOCCalcn/CapAdder1/LKT ==
  SelectedIndex : Inport
  Current100mA : Inport  Port=2
  CellLowTemp : Inport  Port=3
  UCell : Inport  Port=4
  SOH : Inport  Port=5
  DefaultCap : Inport  Port=6
  Enable : EnablePort
  Add : Sum  AccumDataTypeStr=int32  OutDataTypeStr=int32
  Add1 : Sum  Inputs=+-  OutDataTypeStr=int32
  Constant : Constant  OutDataTypeStr=uint8
  Constant1 : Constant  Value=SOC_SOHResolution  OutDataTypeStr=uint16
  Constant10 : Constant  Value=SOC_SOCResolution  OutDataTypeStr=uint16
  Constant12 : Constant  Value=2  OutDataTypeStr=uint8
  Constant13 : Constant  Value=3  OutDataTypeStr=uint8
  Constant17 : Constant  Value=SOC_CapTemp_HLimit  OutDataTypeStr=uint8
  Constant18 : Constant  Value=SOC_MaxCap_AmS
  Constant2 : Constant  Value=8000
  Constant22 : Constant  Value=2  OutDataTypeStr=uint16
  Constant23 : Constant  Value=0  OutDataTypeStr=uint16
  Constant5 : Constant  Value=SOC_MaxCap_AmS
  Constant6 : Constant  Value=SOC_MaxCap_AmS
  Constant7 : Constant  Value=SOC_NominalCap_AmS
  Constant8 : Constant  Value=SOC_SOHResolution  OutDataTypeStr=uint16
  Constant9 : Constant  Value=SOC_CapTemp_LLimit  OutDataTypeStr=uint8
  Divide1 : Product  Inputs=*/*  OutDataTypeStr=uint32
  Divide10 : Product  Inputs=**  OutDataTypeStr=uint32
  Divide2 : Product  Inputs=**  OutDataTypeStr=uint32
  Divide3 : Product  Inputs=*/  OutDataTypeStr=uint32
  Divide4 : Product  Inputs=*/*  OutDataTypeStr=uint32
  Interval Test Dynamic : simulink/Logic and Bit Operations/Interval Test Dynamic  IntervalClosedRight=off  IntervalClosedLeft=off  OutDataTypeStr=boolean
      settings: SourceProductName=Simulink  SourceProductBaseCode=SL
  LKT_Temp20 : Subsystem
  LKT_Temp40 : Subsystem
  LKT_Temp45 : Subsystem
  LeftCap1 : MultiPortSwitch  DataPortOrder=Specify indices  Inputs={1,2,3}
  Logical Operator2 : Logic  Operator=NOT  AllPortsSameDT=off  OutDataTypeStr=boolean
  Relational Operator : RelationalOperator  Operator===  OutDataTypeStr=boolean  RndMeth=Simplest
  Relational Operator1 : RelationalOperator  Operator===  OutDataTypeStr=boolean  RndMeth=Simplest
  Relational Operator2 : RelationalOperator  Operator===  OutDataTypeStr=boolean  RndMeth=Simplest
  Relational Operator3 : RelationalOperator  OutDataTypeStr=boolean  RndMeth=Simplest
  Saturation Dynamic : simulink/Discontinuities/Saturation Dynamic  OutMin=[]  OutMax=[]  OutDataTypeStr=uint32  OutputDataTypeScalingMode=uint32  OutDataType=fixdt(1, 16)  OutScaling=2^-10  DoSatur=off
  Switch : Switch  Criteria=u2 > Threshold
  Switch3 : Switch  Criteria=u2 > Threshold
  TempCapTable1 : Lookup_n-D  NumberOfTableDimensions=1  BreakpointsForDimension1=SOC_TempCap_TempBuffer  Table=SOC_TempCap_CapBuffer  ExtrapMethod=Clip  InternalRulePriority=Speed  OutDataTypeStr=uint16  RndMeth=Simplest  InputSameDT=on
  LeftCap : Outport
  wires:
  Divide10/1 -> Saturation Dynamic/1
  Constant22/1 -> Divide10/2
  Constant9/1 -> Interval Test Dynamic/3
  Constant5/1 -> Divide10/1
  Constant10/1 -> Divide1/2
  Logical Operator2/1 -> Switch3/2
  Divide2/1 -> Switch3/3
  Interval Test Dynamic/1 -> Logical Operator2/1
  LeftCap1/1 -> Relational Operator3/1, Divide1/3  "soc"
  Add/1 -> Saturation Dynamic/2
  Constant6/1 -> Add1/1
  Constant23/1 -> Saturation Dynamic/3
  Switch3/1 -> Add1/2, Divide1/1  "Qt"
  Constant8/1 -> Divide4/2
  Divide4/1 -> Add/2
  Switch/1 -> LeftCap/1
  SOH/1 -> Divide4/3
  Divide1/1 -> Divide4/1  "当前可用剩余容量"
  Constant1/1 -> Divide3/2
  CellLowTemp/1 -> Interval Test Dynamic/2, TempCapTable1/1
  Constant18/1 -> Switch3/1
  Add1/1 -> Add/1  "TempDeltaCap"
  Divide3/1 -> Divide2/2
  Constant7/1 -> Divide3/1
  Constant17/1 -> Interval Test Dynamic/1
  TempCapTable1/1 -> Divide2/1
  SelectedIndex/1 -> Relational Operator1/1, Relational Operator2/1, Relational Operator/1, LeftCap1/1
  Constant/1 -> Relational Operator/2
  Relational Operator/1 -> LKT_Temp20/Enable
  Current100mA/1 -> LKT_Temp45/1(Cur), LKT_Temp40/1(Cur), LKT_Temp20/1(Cur)
  Constant12/1 -> Relational Operator1/2
  Relational Operator1/1 -> LKT_Temp40/Enable
  Relational Operator2/1 -> LKT_Temp45/Enable
  Constant13/1 -> Relational Operator2/2
  UCell/1 -> LKT_Temp45/2(UCell), LKT_Temp40/2(UCell), LKT_Temp20/2(UCell)
  LKT_Temp20/1(SOC) -> LeftCap1/2
  LKT_Temp40/1(SOC) -> LeftCap1/3  "Temp40SOC"
  LKT_Temp45/1(SOC) -> LeftCap1/4
  Constant2/1 -> Relational Operator3/2
  Relational Operator3/1 -> Switch/2
  Saturation Dynamic/1 -> Switch/1
  DefaultCap/1 -> Switch/3
